simulink library "rewardLibrary"  (R2022b)
settings: Solver=VariableStepAuto  StartTime=0.0  StopTime=10.0  RelTol=1e-3
values from neighbouring files (symbols this model uses):
  accel_vec = (-4:0.5:4)'    [setUpModel.m]
  Ts = 0.1    [setUpMPC.m]
  TsRL = Ts    [setUpRLEnv.m]
  vel_vec = 0:2:20    [setUpModel.m]
undefined symbols (not defined in the file or in its folder): A, B, C, curvature1, D, D_default, DiscIntNeverNeededParam, E, F, gradbp1, k_sigmoid, steer_lim, t_gap, v_set, x_colpen, y_colpen, Z_colpen
libraries: simulink x379, $bdroot x2, mpcadaslib x1
(part 1 of 9)
settings Model: Creator=16koc1  LastModifiedBy=16koc1

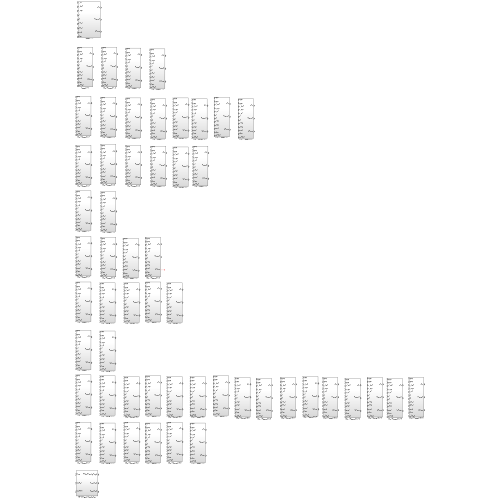
[thumbnail: Simulink's stored preview of the top-level diagram]
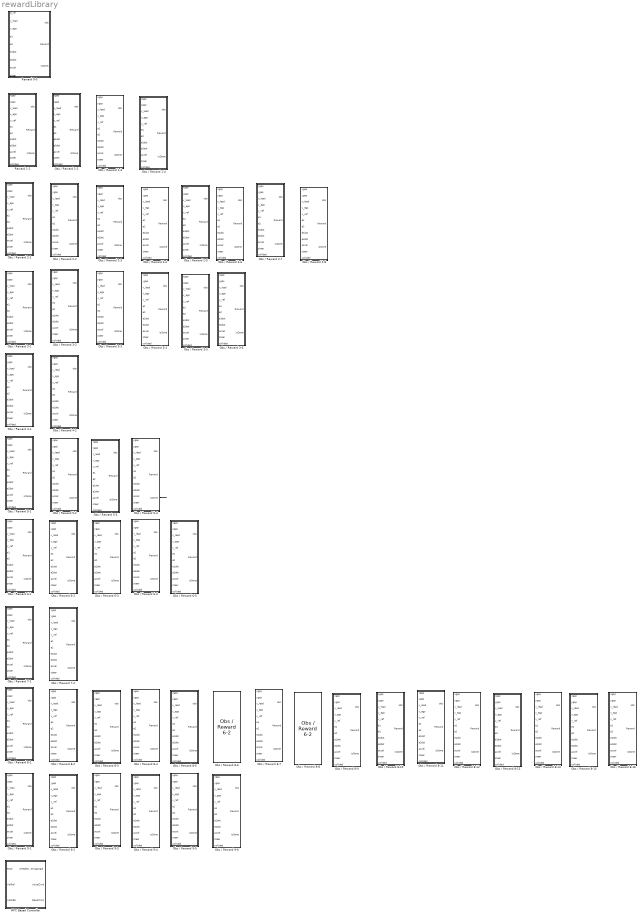
== system rewardLibrary ==
  MPC Based Controller : Subsystem  VariantControl=Stanley
  Obs / Reward 1-2 : Subsystem
  Obs / Reward 1-3 : Subsystem
  Obs / Reward 1-4 : Subsystem
  Obs / Reward 2-1 : Subsystem
  Obs / Reward 2-2 : Subsystem
  Obs / Reward 2-3 : Subsystem
  Obs / Reward 2-4 : Subsystem
  Obs / Reward 2-5 : Subsystem
  Obs / Reward 2-6 : Subsystem
  Obs / Reward 2-7 : Subsystem
  Obs / Reward 2-8 : Subsystem
  Obs / Reward 3-1 : Subsystem
  Obs / Reward 3-2 : Subsystem
  Obs / Reward 3-3 : Subsystem
  Obs / Reward 3-4 : Subsystem
  Obs / Reward 3-5 : Subsystem
  Obs / Reward 3-6 : Subsystem
  Obs / Reward 4-1 : Subsystem
  Obs / Reward 4-2 : Subsystem
  Obs / Reward 5-1 : Subsystem
  Obs / Reward 5-2 : Subsystem
  Obs / Reward 5-3 : Subsystem
  Obs / Reward 5-4 : Subsystem
  Obs / Reward 6-1 : Subsystem  AncestorBlock=rewardLibrary/Obs // Reward 5-3
      settings: LibrarySourceBlock=rewardLibrary/Obs // Reward 5-3
  Obs / Reward 6-2 : Subsystem  AncestorBlock=rewardLibrary/Obs // Reward 5-3
      settings: LibrarySourceBlock=rewardLibrary/Obs // Reward 6-2
  Obs / Reward 6-3 : Subsystem  AncestorBlock=rewardLibrary/Obs // Reward 5-3
      settings: LibrarySourceBlock=rewardLibrary/Obs // Reward 5-3
  Obs / Reward 6-4 : Subsystem  AncestorBlock=rewardLibrary/Obs // Reward 6-2
      settings: LibrarySourceBlock=rewardLibrary/Obs // Reward 6-2
  Obs / Reward 6-5 : Subsystem  AncestorBlock=rewardLibrary/Obs // Reward 6-2
      settings: LibrarySourceBlock=rewardLibrary/Obs // Reward 6-2
  Obs / Reward 7-1 : Subsystem  AncestorBlock=rewardLibrary/Obs // Reward 6-2
      settings: LibrarySourceBlock=rewardLibrary/Obs // Reward 6-2
  Obs / Reward 7-2 : Subsystem  AncestorBlock=rewardLibrary/Obs // Reward 6-2
      settings: LibrarySourceBlock=rewardLibrary/Obs // Reward 6-2
  Obs / Reward 8-1 : Subsystem  AncestorBlock=rewardLibrary/Obs // Reward 6-2
      settings: LibrarySourceBlock=rewardLibrary/Obs // Reward 6-2
  Obs / Reward 8-10 : Subsystem  AncestorBlock=rewardLibrary/Obs // Reward 6-2
      settings: LibrarySourceBlock=rewardLibrary/Obs // Reward 6-2
  Obs / Reward 8-11 : Subsystem  AncestorBlock=rewardLibrary/Obs // Reward 6-2
      settings: LibrarySourceBlock=rewardLibrary/Obs // Reward 6-2
  Obs / Reward 8-12 : Subsystem  AncestorBlock=rewardLibrary/Obs // Reward 6-2
      settings: LibrarySourceBlock=rewardLibrary/Obs // Reward 6-2
  Obs / Reward 8-13 : Subsystem  AncestorBlock=rewardLibrary/Obs // Reward 6-2
      settings: LibrarySourceBlock=rewardLibrary/Obs // Reward 6-2
  Obs / Reward 8-14 : Subsystem  AncestorBlock=rewardLibrary/Obs // Reward 6-2
      settings: LibrarySourceBlock=rewardLibrary/Obs // Reward 6-2
  Obs / Reward 8-15 : Subsystem  AncestorBlock=rewardLibrary/Obs // Reward 6-2
      settings: LibrarySourceBlock=rewardLibrary/Obs // Reward 6-2
  Obs / Reward 8-16 : Subsystem  AncestorBlock=rewardLibrary/Obs // Reward 6-2
      settings: LibrarySourceBlock=rewardLibrary/Obs // Reward 6-2
  Obs / Reward 8-2 : Subsystem  AncestorBlock=rewardLibrary/Obs // Reward 6-2
      settings: LibrarySourceBlock=rewardLibrary/Obs // Reward 6-2
  Obs / Reward 8-3 : Subsystem  AncestorBlock=rewardLibrary/Obs // Reward 6-2
      settings: LibrarySourceBlock=rewardLibrary/Obs // Reward 6-2
  Obs / Reward 8-4 : Subsystem  AncestorBlock=rewardLibrary/Obs // Reward 6-2
      settings: LibrarySourceBlock=rewardLibrary/Obs // Reward 6-2
  Obs / Reward 8-5 : Subsystem  AncestorBlock=rewardLibrary/Obs // Reward 6-2
      settings: LibrarySourceBlock=rewardLibrary/Obs // Reward 6-2
  Obs / Reward 8-6 : $bdroot/Obs // Reward 6-2  SystemSampleTime=-1  VariantActivationTime=update diagram  Latency=0  AutoFrameSizeCalculation=off
  Obs / Reward 8-7 : Subsystem  AncestorBlock=rewardLibrary/Obs // Reward 6-2
      settings: LibrarySourceBlock=rewardLibrary/Obs // Reward 6-2
  Obs / Reward 8-8 : $bdroot/Obs // Reward 6-2  SystemSampleTime=-1  VariantActivationTime=update diagram  Latency=0  AutoFrameSizeCalculation=off
      link override A: Gain=0
      link override Path following/Gain11: Gain=-0.006
      link override Path following/Gain4: Gain=-0.9
  Obs / Reward 8-9 : Subsystem  AncestorBlock=rewardLibrary/Obs // Reward 6-2
      settings: LibrarySourceBlock=rewardLibrary/Obs // Reward 6-2
  Obs / Reward 9-1 : Subsystem  AncestorBlock=rewardLibrary/Obs // Reward 6-2
      settings: LibrarySourceBlock=rewardLibrary/Obs // Reward 6-2
  Obs / Reward 9-2 : Subsystem  AncestorBlock=rewardLibrary/Obs // Reward 6-2
      settings: LibrarySourceBlock=rewardLibrary/Obs // Reward 6-2
  Obs / Reward 9-3 : Subsystem  AncestorBlock=rewardLibrary/Obs // Reward 6-2
      settings: LibrarySourceBlock=rewardLibrary/Obs // Reward 6-2
  Obs / Reward 9-4 : Subsystem  AncestorBlock=rewardLibrary/Obs // Reward 6-2
      settings: LibrarySourceBlock=rewardLibrary/Obs // Reward 6-2
  Obs / Reward 9-5 : Subsystem  AncestorBlock=rewardLibrary/Obs // Reward 6-2
      settings: LibrarySourceBlock=rewardLibrary/Obs // Reward 6-2
  Obs / Reward 9-6 : Subsystem  AncestorBlock=rewardLibrary/Obs // Reward 6-2
      settings: LibrarySourceBlock=rewardLibrary/Obs // Reward 6-2
  Reward 0-0 : Subsystem
  Reward 1-1 : Subsystem
  wires:
  Obs / Reward 5-4/3(isDone) -> ?

== system rewardLibrary/MPC Based Controller ==
  note: This 2-D Lookup Table was created using a for-loop and then normalizing. This is required because the output of the MPC controller is acceleration (m/s^2), but the powertrain model uses pedal commands from 0-1.
      |
      | Here are the steps in the script to create the table:
      |
      | 1.) The for-loop is used to calculate the required torque (Nm) from the powertrain.
      |
      | 2.) The positive torque values are normalized based on peak positive motor torque, and the negative torques are normalized based on the peak brake pressure. This results in a pedal map with values of -1 to 1.
      |
      | This map required two values to be calibrated.
      |
      | This is a simple linearized map, but this can be altered for better drivability.
  note: The 'Dead Zone' blocks is used to ensure that the pedal command is zero.
  note: This block comes from the "Lane Keeping Assist System Using Model Predictive Control" example.
  Pose : Inport
  VelRef : Inport  Port=2
  VelFdbk : Inport  Port=3
  1-D Lookup Table1 : Lookup_n-D  NumberOfTableDimensions=1  BreakpointsForDimension1=gradbp1  Table=curvature1  InterpMethod=Cubic spline  ExtrapMethod=Clip  InternalRulePriority=Speed  RndMeth=Simplest
  Integrator : Integrator
  Path Following Control System MPC : mpcadaslib/Path Following Control System  VariantControl=Variant2  ModelType=Use vehicle parameters  VehicleMass=2000  VehicleYawInertia=4000  LengthToFront=1.4  LengthToRear=1.6  FrontTireStiffness=12e3  RearTireStiffness=11e3  AccelTimeConstant=0.5  EgoModelMatrixA=[-2,zeros(1,3);1,zeros(1,3);zeros(1,2),-4.4021,-12.4603;zeros(1,2),1.3913,-5.1868]  EgoModelMatrixB=[2,zeros(1,3);zeros(1,2),24.1270,15.8609]'  EgoModelMatrixC=[zeros(3,1),eye(3)]  InitialLongVel=v_o1  TransportLag=0  spaceCtrl=off  DefaultSpacing=10  MinSteering=umin  umin_ext=off  MaxSteering=umax  umax_ext=off  MinAcceleration=amin  amin_ext=off  MaxAcceleration=amax  amax_ext=off  Ts=Ts  PredictionHorizon=pred_horizon  ControlHorizon=cont_horizon  LongWeight=w_veltrack  LateralWeight=w_laterror  AccelRateWeight=w_dax  SteerRateWeight=w_dphi  suboptimal=off  maxiter=10  datatypeopt=double  optmode=off  trackmode=off
      link override Longitudinal velocity must be positive: enabled=on
  Pedal map : Subsystem
  Sensor Dynamics : Subsystem
  Terminator : Terminator
  WheelSteeringAngle : Outport
  AccelCmd : Outport  Port=2
  DecelCmd : Outport  Port=3
  wires:
  Integrator/1 -> 1-D Lookup Table1/1
  [ydot1] -> Sensor Dynamics/3(Lateral velocity)
  [yawrate1] -> Sensor Dynamics/4(Yaw rate)
  VelFdbk/1 -> Sensor Dynamics/2(Longitudinal velocity), Path Following Control System MPC/2, Pedal map/1(vx), Integrator/1  "vx"
  VelRef/1 -> Path Following Control System MPC/1
  Pose/1 -> Terminator/1
  Path Following Control System MPC/2 -> WheelSteeringAngle/1
  Path Following Control System MPC/1 -> Pedal map/2(a)  "a"
  Pedal map/1(Out1) -> AccelCmd/1
  Pedal map/2(Out2) -> DecelCmd/1
  Sensor Dynamics/2(Relative yaw angle) -> Path Following Control System MPC/5
  Sensor Dynamics/1(Lateral deviation) -> Path Following Control System MPC/4
  1-D Lookup Table1/1 -> Sensor Dynamics/1(Current curvature), Path Following Control System MPC/3

== system rewardLibrary/Obs // Reward 1-2 ==
  xgap : Inport
  ygap : Inport  Port=2
  v_lead : Inport  Port=3
  v_ego : Inport  Port=4
  v_ref : Inport  Port=5
  e1 : Inport  Port=6
  e2 : Inport  Port=7
  e1dot : Inport  Port=8
  e2dot : Inport  Port=9
  accel : Inport  Port=10
  steer : Inport  Port=11
  collided : Inport  Port=12
  Abs : Abs  SaturateOnIntegerOverflow=off
  Compare To Constant : simulink/Logic and Bit Operations/Compare To Constant  relop=<=  const=6  OutDataTypeStr=boolean
  Gain : Gain  Gain=10
  Subsystem : Subsystem
  Subsystem1 : Subsystem
  Subsystem2 : Subsystem
  Sum : Sum  Inputs=-+|
  Terminator{,1..3} (4 alike) : Terminator
  obs : Outport  VectorParamsAs1DForOutWhenUnconnected=off
  Reward : Outport  Port=2  VectorParamsAs1DForOutWhenUnconnected=off
  isDone : Outport  Port=3  VectorParamsAs1DForOutWhenUnconnected=off
  tag scope: onTrack=global
  wires:
  e2dot/1 -> Subsystem/6(e2dot)
  e1/1 -> Abs/1, Subsystem/3(e1), Subsystem2/2(e1), Subsystem1/2(e1)
  e2/1 -> Subsystem2/3(e2), Subsystem/4(e2)
  v_ego/1 -> Subsystem2/1(v_ego), Subsystem/1(v_ego)
  Subsystem2/1(isDone) -> Gain/1, isDone/1
  Subsystem/2(v_err) -> Subsystem1/3(v_err)
  v_lead/1 -> Terminator/1
  xgap/1 -> Terminator1/1
  steer/1 -> Subsystem1/1(steer)
  Subsystem/1(obs) -> obs/1
  e1dot/1 -> Subsystem/5(e1dot)
  Subsystem1/1(reward) -> Sum/2
  Sum/1 -> Reward/1
  Gain/1 -> Sum/1
  Abs/1 -> Compare To Constant/1
  Compare To Constant/1 -> [onTrack]
  collided/1 -> Terminator3/1
  v_ref/1 -> Subsystem/2(v_ref)
  ygap/1 -> Terminator2/1
  accel/1 -> Subsystem1/4(accel)

== system rewardLibrary/Obs // Reward 1-3 ==
  xgap : Inport
  ygap : Inport  Port=2
  v_lead : Inport  Port=3
  v_ego : Inport  Port=4
  v_ref : Inport  Port=5
  e1 : Inport  Port=6
  e2 : Inport  Port=7
  e1dot : Inport  Port=8
  e2dot : Inport  Port=9
  accel : Inport  Port=10
  steer : Inport  Port=11
  collided : Inport  Port=12
  Abs : Abs  SaturateOnIntegerOverflow=off
  Compare To Constant : simulink/Logic and Bit Operations/Compare To Constant  relop=<=  const=6  OutDataTypeStr=boolean
  Gain : Gain  Gain=300
  Subsystem : Subsystem
  Subsystem1 : Subsystem
  Subsystem2 : Subsystem
  Sum : Sum  Inputs=-+|
  Terminator{,1..3} (4 alike) : Terminator
  obs : Outport  VectorParamsAs1DForOutWhenUnconnected=off
  Reward : Outport  Port=2  VectorParamsAs1DForOutWhenUnconnected=off
  isDone : Outport  Port=3  VectorParamsAs1DForOutWhenUnconnected=off
  tag scope: onTrack=global
  wires:
  e2dot/1 -> Subsystem/6(e2dot)
  e1/1 -> Abs/1, Subsystem/3(e1), Subsystem2/2(e1), Subsystem1/2(e1)
  e2/1 -> Subsystem2/3(e2), Subsystem/4(e2)
  v_ego/1 -> Subsystem2/1(v_ego), Subsystem/1(v_ego)
  Subsystem2/1(isDone) -> Gain/1, isDone/1
  Subsystem/2(v_err) -> Subsystem1/3(v_err)
  v_lead/1 -> Terminator/1
  xgap/1 -> Terminator1/1
  steer/1 -> Subsystem1/1(steer)
  Subsystem/1(obs) -> obs/1
  e1dot/1 -> Subsystem/5(e1dot)
  Subsystem1/1(reward) -> Sum/2
  Sum/1 -> Reward/1
  Gain/1 -> Sum/1
  Abs/1 -> Compare To Constant/1
  Compare To Constant/1 -> [onTrack]
  collided/1 -> Terminator3/1
  v_ref/1 -> Subsystem/2(v_ref)
  ygap/1 -> Terminator2/1
  accel/1 -> Subsystem1/4(accel)

== system rewardLibrary/Obs // Reward 1-4 ==
  xgap : Inport
  ygap : Inport  Port=2
  v_lead : Inport  Port=3
  v_ego : Inport  Port=4
  v_ref : Inport  Port=5
  e1 : Inport  Port=6
  e2 : Inport  Port=7
  e1dot : Inport  Port=8
  e2dot : Inport  Port=9
  accel : Inport  Port=10
  steer : Inport  Port=11
  collided : Inport  Port=12
  Abs : Abs  SaturateOnIntegerOverflow=off
  Compare To Constant : simulink/Logic and Bit Operations/Compare To Constant  relop=<=  const=6  OutDataTypeStr=boolean
  Gain : Gain  Gain=100
  Subsystem : Subsystem
  Subsystem1 : Subsystem
  Subsystem2 : Subsystem
  Sum : Sum  Inputs=-+|
  Terminator{,1..3} (4 alike) : Terminator
  obs : Outport  VectorParamsAs1DForOutWhenUnconnected=off
  Reward : Outport  Port=2  VectorParamsAs1DForOutWhenUnconnected=off
  isDone : Outport  Port=3  VectorParamsAs1DForOutWhenUnconnected=off
  tag scope: onTrack=global
  wires:
  e2dot/1 -> Subsystem/6(e2dot)
  e1/1 -> Abs/1, Subsystem/3(e1), Subsystem2/2(e1), Subsystem1/2(e1)
  e2/1 -> Subsystem2/3(e2), Subsystem/4(e2)
  v_ego/1 -> Subsystem2/1(v_ego), Subsystem/1(v_ego)
  Subsystem2/1(isDone) -> Gain/1, isDone/1
  Subsystem/2(v_err) -> Subsystem1/3(v_err)
  v_lead/1 -> Terminator/1
  xgap/1 -> Terminator1/1
  steer/1 -> Subsystem1/1(steer)
  Subsystem/1(obs) -> obs/1
  e1dot/1 -> Subsystem/5(e1dot)
  Subsystem1/1(reward) -> Sum/2
  Sum/1 -> Reward/1
  Gain/1 -> Sum/1
  Abs/1 -> Compare To Constant/1
  Compare To Constant/1 -> [onTrack]
  collided/1 -> Terminator3/1
  v_ref/1 -> Subsystem/2(v_ref)
  ygap/1 -> Terminator2/1
  accel/1 -> Subsystem1/4(accel)

== system rewardLibrary/Obs // Reward 2-1 ==
  xgap : Inport
  ygap : Inport  Port=2
  v_lead : Inport  Port=3
  v_ego : Inport  Port=4
  v_ref : Inport  Port=5
  e1 : Inport  Port=6
  e2 : Inport  Port=7
  e1dot : Inport  Port=8
  e2dot : Inport  Port=9
  accel : Inport  Port=10
  steer : Inport  Port=11
  collided : Inport  Port=12
  Abs : Abs  SaturateOnIntegerOverflow=off
  Compare To Constant : simulink/Logic and Bit Operations/Compare To Constant  relop=<=  const=6  OutDataTypeStr=boolean
  Gain : Gain  Gain=10
  Subsystem : Subsystem
  Subsystem1 : Subsystem
  Subsystem2 : Subsystem
  Sum : Sum  Inputs=-+|
  Terminator{,1..3} (4 alike) : Terminator
  obs : Outport  VectorParamsAs1DForOutWhenUnconnected=off
  Reward : Outport  Port=2  VectorParamsAs1DForOutWhenUnconnected=off
  isDone : Outport  Port=3  VectorParamsAs1DForOutWhenUnconnected=off
  tag scope: onTrack=global
  wires:
  e2dot/1 -> Subsystem/6(e2dot)
  e1/1 -> Abs/1, Subsystem1/2(e1), Subsystem/3(e1), Subsystem2/2(e1)
  e2/1 -> Subsystem2/3(e2), Subsystem/4(e2)
  v_ego/1 -> Subsystem2/1(v_ego), Subsystem/1(v_ego)
  Subsystem2/1(isDone) -> Gain/1, isDone/1
  v_lead/1 -> Terminator/1
  xgap/1 -> Terminator1/1
  Subsystem/1(obs) -> obs/1
  e1dot/1 -> Subsystem/5(e1dot)
  Sum/1 -> Reward/1
  Gain/1 -> Sum/1
  Abs/1 -> Compare To Constant/1
  Compare To Constant/1 -> [onTrack]
  collided/1 -> Terminator3/1
  v_ref/1 -> Subsystem/2(v_ref)
  ygap/1 -> Terminator2/1
  Subsystem1/1(reward) -> Sum/2
  Subsystem/2(v_err) -> Subsystem1/3(v_err)
  steer/1 -> Subsystem1/1(steer)
  accel/1 -> Subsystem1/4(accel)

== system rewardLibrary/Obs // Reward 2-2 ==
  xgap : Inport
  ygap : Inport  Port=2
  v_lead : Inport  Port=3
  v_ego : Inport  Port=4
  v_ref : Inport  Port=5
  e1 : Inport  Port=6
  e2 : Inport  Port=7
  e1dot : Inport  Port=8
  e2dot : Inport  Port=9
  accel : Inport  Port=10
  steer : Inport  Port=11
  collided : Inport  Port=12
  Abs : Abs  SaturateOnIntegerOverflow=off
  Compare To Constant : simulink/Logic and Bit Operations/Compare To Constant  relop=<=  const=6  OutDataTypeStr=boolean
  Gain : Gain  Gain=10
  Subsystem : Subsystem
  Subsystem1 : Subsystem
  Subsystem2 : Subsystem
  Sum : Sum  Inputs=-+|
  Terminator{,1..3} (4 alike) : Terminator
  obs : Outport  VectorParamsAs1DForOutWhenUnconnected=off
  Reward : Outport  Port=2  VectorParamsAs1DForOutWhenUnconnected=off
  isDone : Outport  Port=3  VectorParamsAs1DForOutWhenUnconnected=off
  tag scope: onTrack=global
  wires:
  e2dot/1 -> Subsystem/6(e2dot)
  e1/1 -> Abs/1, Subsystem1/2(e1), Subsystem/3(e1), Subsystem2/2(e1)
  e2/1 -> Subsystem2/3(e2), Subsystem/4(e2)
  v_ego/1 -> Subsystem2/1(v_ego), Subsystem/1(v_ego)
  Subsystem2/1(isDone) -> Gain/1, isDone/1
  v_lead/1 -> Terminator/1
  xgap/1 -> Terminator1/1
  Subsystem/1(obs) -> obs/1
  e1dot/1 -> Subsystem/5(e1dot)
  Sum/1 -> Reward/1
  Gain/1 -> Sum/1
  Abs/1 -> Compare To Constant/1
  Compare To Constant/1 -> [onTrack]
  collided/1 -> Terminator3/1
  v_ref/1 -> Subsystem/2(v_ref)
  ygap/1 -> Terminator2/1
  Subsystem1/1(reward) -> Sum/2
  Subsystem/2(v_err) -> Subsystem1/3(v_err)
  steer/1 -> Subsystem1/1(steer)
  accel/1 -> Subsystem1/4(accel)

== system rewardLibrary/Obs // Reward 2-3 ==
  xgap : Inport
  ygap : Inport  Port=2
  v_lead : Inport  Port=3
  v_ego : Inport  Port=4
  v_ref : Inport  Port=5
  e1 : Inport  Port=6
  e2 : Inport  Port=7
  e1dot : Inport  Port=8
  e2dot : Inport  Port=9
  accel : Inport  Port=10
  steer : Inport  Port=11
  collided : Inport  Port=12
  Abs : Abs  SaturateOnIntegerOverflow=off
  Compare To Constant : simulink/Logic and Bit Operations/Compare To Constant  relop=<=  const=6  OutDataTypeStr=boolean
  Gain : Gain  Gain=10
  Gain1 : Gain  Gain=100
  OR : Logic  Operator=OR  IconShape=distinctive  AllPortsSameDT=off  OutDataTypeStr=boolean
  Subsystem : Subsystem
  Subsystem1 : Subsystem
  Subsystem2 : Subsystem
  Sum : Sum  Inputs=--+
  Terminator{,1..3} (4 alike) : Terminator
  obs : Outport  VectorParamsAs1DForOutWhenUnconnected=off
  Reward : Outport  Port=2  VectorParamsAs1DForOutWhenUnconnected=off
  isDone : Outport  Port=3  VectorParamsAs1DForOutWhenUnconnected=off
  tag scope: onTrack=global
  wires:
  e2dot/1 -> Subsystem/6(e2dot)
  e1/1 -> Abs/1, Subsystem1/2(e1), Subsystem/3(e1), Subsystem2/2(e1)
  e2/1 -> Subsystem2/3(e2), Subsystem/4(e2)
  v_ego/1 -> Subsystem2/1(v_ego), Subsystem/1(v_ego)
  Subsystem2/1(isDone) -> OR/1, Gain/1
  v_lead/1 -> Terminator/1
  xgap/1 -> Terminator1/1
  Subsystem/1(obs) -> obs/1
  e1dot/1 -> Subsystem/5(e1dot)
  Sum/1 -> Reward/1
  Gain/1 -> Sum/1
  Abs/1 -> Compare To Constant/1
  Compare To Constant/1 -> [onTrack]
  collided/1 -> Terminator3/1
  v_ref/1 -> Subsystem/2(v_ref)
  ygap/1 -> Terminator2/1
  Subsystem1/1(reward) -> Sum/3
  Subsystem/2(v_err) -> Subsystem1/3(v_err)
  steer/1 -> Subsystem1/1(steer)
  accel/1 -> Subsystem1/4(accel)
  OR/1 -> isDone/1
  Subsystem2/2(spinTurn) -> Gain1/1, OR/2
  Gain1/1 -> Sum/2

== system rewardLibrary/Obs // Reward 2-4 ==
  xgap : Inport
  ygap : Inport  Port=2
  v_lead : Inport  Port=3
  v_ego : Inport  Port=4
  v_ref : Inport  Port=5
  e1 : Inport  Port=6
  e2 : Inport  Port=7
  e1dot : Inport  Port=8
  e2dot : Inport  Port=9
  accel : Inport  Port=10
  steer : Inport  Port=11
  collided : Inport  Port=12
  Abs : Abs  SaturateOnIntegerOverflow=off
  Compare To Constant : simulink/Logic and Bit Operations/Compare To Constant  relop=<=  const=6  OutDataTypeStr=boolean
  Gain : Gain  Gain=10
  Gain1 : Gain  Gain=100
  OR : Logic  Operator=OR  IconShape=distinctive  AllPortsSameDT=off  OutDataTypeStr=boolean
  Subsystem : Subsystem
  Subsystem1 : Subsystem
  Subsystem2 : Subsystem
  Sum : Sum  Inputs=--+
  Terminator{,1..3} (4 alike) : Terminator
  obs : Outport  VectorParamsAs1DForOutWhenUnconnected=off
  Reward : Outport  Port=2  VectorParamsAs1DForOutWhenUnconnected=off
  isDone : Outport  Port=3  VectorParamsAs1DForOutWhenUnconnected=off
  tag scope: onTrack=global
  wires:
  e2dot/1 -> Subsystem/6(e2dot)
  e1/1 -> Abs/1, Subsystem1/2(e1), Subsystem/3(e1), Subsystem2/2(e1)
  e2/1 -> Subsystem2/3(e2), Subsystem/4(e2)
  v_ego/1 -> Subsystem2/1(v_ego), Subsystem/1(v_ego)
  Subsystem2/1(isDone) -> OR/1, Gain/1
  v_lead/1 -> Terminator/1
  xgap/1 -> Terminator1/1
  Subsystem/1(obs) -> obs/1
  e1dot/1 -> Subsystem/5(e1dot)
  Sum/1 -> Reward/1
  Gain/1 -> Sum/1
  Abs/1 -> Compare To Constant/1
  Compare To Constant/1 -> [onTrack]
  collided/1 -> Terminator3/1
  v_ref/1 -> Subsystem/2(v_ref)
  ygap/1 -> Terminator2/1
  Subsystem1/1(reward) -> Sum/3
  Subsystem/2(v_err) -> Subsystem1/3(v_err)
  steer/1 -> Subsystem1/1(steer)
  accel/1 -> Subsystem1/4(accel)
  OR/1 -> isDone/1
  Subsystem2/2(spinTurn) -> Gain1/1, OR/2
  Gain1/1 -> Sum/2

== system rewardLibrary/Obs // Reward 2-5 ==
  xgap : Inport
  ygap : Inport  Port=2
  v_lead : Inport  Port=3
  v_ego : Inport  Port=4
  v_ref : Inport  Port=5
  e1 : Inport  Port=6
  e2 : Inport  Port=7
  e1dot : Inport  Port=8
  e2dot : Inport  Port=9
  accel : Inport  Port=10
  steer : Inport  Port=11
  collided : Inport  Port=12
  Abs : Abs  SaturateOnIntegerOverflow=off
  Compare To Constant : simulink/Logic and Bit Operations/Compare To Constant  relop=<=  const=6  OutDataTypeStr=boolean
  Gain : Gain  Gain=10
  Gain1 : Gain  Gain=100
  OR : Logic  Operator=OR  IconShape=distinctive  AllPortsSameDT=off  OutDataTypeStr=boolean
  Subsystem : Subsystem
  Subsystem1 : Subsystem
  Subsystem2 : Subsystem
  Sum : Sum  Inputs=--+
  Terminator{,1..3} (4 alike) : Terminator
  obs : Outport  VectorParamsAs1DForOutWhenUnconnected=off
  Reward : Outport  Port=2  VectorParamsAs1DForOutWhenUnconnected=off
  isDone : Outport  Port=3  VectorParamsAs1DForOutWhenUnconnected=off
  tag scope: onTrack=global
  wires:
  e2dot/1 -> Subsystem/6(e2dot)
  e1/1 -> Abs/1, Subsystem1/2(e1), Subsystem/3(e1), Subsystem2/2(e1)
  e2/1 -> Subsystem2/3(e2), Subsystem/4(e2)
  v_ego/1 -> Subsystem2/1(v_ego), Subsystem/1(v_ego)
  Subsystem2/1(isDone) -> OR/1, Gain/1
  v_lead/1 -> Terminator/1
  xgap/1 -> Terminator1/1
  Subsystem/1(obs) -> obs/1
  e1dot/1 -> Subsystem/5(e1dot)
  Sum/1 -> Reward/1
  Gain/1 -> Sum/1
  Abs/1 -> Compare To Constant/1
  Compare To Constant/1 -> [onTrack]
  collided/1 -> Terminator3/1
  v_ref/1 -> Subsystem/2(v_ref)
  ygap/1 -> Terminator2/1
  Subsystem1/1(reward) -> Sum/3
  Subsystem/2(v_err) -> Subsystem1/3(v_err)
  steer/1 -> Subsystem1/1(steer)
  accel/1 -> Subsystem1/4(accel)
  OR/1 -> isDone/1
  Subsystem2/2(spinTurn) -> Gain1/1, OR/2
  Gain1/1 -> Sum/2

== system rewardLibrary/Obs // Reward 2-6 ==
  xgap : Inport
  ygap : Inport  Port=2
  v_lead : Inport  Port=3
  v_ego : Inport  Port=4
  v_ref : Inport  Port=5
  e1 : Inport  Port=6
  e2 : Inport  Port=7
  e1dot : Inport  Port=8
  e2dot : Inport  Port=9
  accel : Inport  Port=10
  steer : Inport  Port=11
  collided : Inport  Port=12
  Abs : Abs  SaturateOnIntegerOverflow=off
  Compare To Constant : simulink/Logic and Bit Operations/Compare To Constant  relop=<=  const=6  OutDataTypeStr=boolean
  Gain : Gain  Gain=10
  Gain1 : Gain  Gain=100
  OR : Logic  Operator=OR  IconShape=distinctive  AllPortsSameDT=off  OutDataTypeStr=boolean
  Subsystem : Subsystem
  Subsystem1 : Subsystem
  Subsystem2 : Subsystem
  Sum : Sum  Inputs=--+
  Terminator{,1..3} (4 alike) : Terminator
  obs : Outport  VectorParamsAs1DForOutWhenUnconnected=off
  Reward : Outport  Port=2  VectorParamsAs1DForOutWhenUnconnected=off
  isDone : Outport  Port=3  VectorParamsAs1DForOutWhenUnconnected=off
  tag scope: onTrack=global
  wires:
  e2dot/1 -> Subsystem/6(e2dot)
  e1/1 -> Abs/1, Subsystem1/2(e1), Subsystem/3(e1), Subsystem2/2(e1)
  e2/1 -> Subsystem2/3(e2), Subsystem/4(e2)
  v_ego/1 -> Subsystem2/1(v_ego), Subsystem/1(v_ego)
  Subsystem2/1(isDone) -> OR/1, Gain/1
  v_lead/1 -> Terminator/1
  xgap/1 -> Terminator1/1
  Subsystem/1(obs) -> obs/1
  e1dot/1 -> Subsystem/5(e1dot)
  Sum/1 -> Reward/1
  Gain/1 -> Sum/1
  Abs/1 -> Compare To Constant/1
  Compare To Constant/1 -> [onTrack]
  collided/1 -> Terminator3/1
  v_ref/1 -> Subsystem/2(v_ref)
  ygap/1 -> Terminator2/1
  Subsystem1/1(reward) -> Sum/3
  Subsystem/2(v_err) -> Subsystem1/3(v_err)
  steer/1 -> Subsystem1/1(steer)
  accel/1 -> Subsystem1/4(accel)
  OR/1 -> isDone/1
  Subsystem2/2(spinTurn) -> Gain1/1, OR/2
  Gain1/1 -> Sum/2

== system rewardLibrary/Obs // Reward 2-7 ==
  xgap : Inport
  ygap : Inport  Port=2
  v_lead : Inport  Port=3
  v_ego : Inport  Port=4
  v_ref : Inport  Port=5
  e1 : Inport  Port=6
  e2 : Inport  Port=7
  e1dot : Inport  Port=8
  e2dot : Inport  Port=9
  accel : Inport  Port=10
  steer : Inport  Port=11
  collided : Inport  Port=12
  Abs : Abs  SaturateOnIntegerOverflow=off
  Compare To Constant : simulink/Logic and Bit Operations/Compare To Constant  relop=<=  const=6  OutDataTypeStr=boolean
  Gain : Gain  Gain=10
  Gain1 : Gain  Gain=100
  OR : Logic  Operator=OR  IconShape=distinctive  AllPortsSameDT=off  OutDataTypeStr=boolean
  Subsystem : Subsystem
  Subsystem1 : Subsystem
  Subsystem2 : Subsystem
  Sum : Sum  Inputs=--+
  Terminator{,1..3} (4 alike) : Terminator
  obs : Outport  VectorParamsAs1DForOutWhenUnconnected=off
  Reward : Outport  Port=2  VectorParamsAs1DForOutWhenUnconnected=off
  isDone : Outport  Port=3  VectorParamsAs1DForOutWhenUnconnected=off
  tag scope: onTrack=global
  wires:
  e2dot/1 -> Subsystem/6(e2dot)
  e1/1 -> Abs/1, Subsystem1/2(e1), Subsystem/3(e1), Subsystem2/2(e1)
  e2/1 -> Subsystem2/3(e2), Subsystem/4(e2)
  v_ego/1 -> Subsystem2/1(v_ego), Subsystem/1(v_ego)
  Subsystem2/1(isDone) -> OR/1, Gain/1
  v_lead/1 -> Terminator/1
  xgap/1 -> Terminator1/1
  Subsystem/1(obs) -> obs/1
  e1dot/1 -> Subsystem/5(e1dot)
  Sum/1 -> Reward/1
  Gain/1 -> Sum/1
  Abs/1 -> Compare To Constant/1
  Compare To Constant/1 -> [onTrack]
  collided/1 -> Terminator3/1
  v_ref/1 -> Subsystem/2(v_ref)
  ygap/1 -> Terminator2/1
  Subsystem1/1(reward) -> Sum/3
  Subsystem/2(v_err) -> Subsystem1/3(v_err)
  steer/1 -> Subsystem1/1(steer)
  accel/1 -> Subsystem1/4(accel)
  OR/1 -> isDone/1
  Subsystem2/2(spinTurn) -> Gain1/1, OR/2
  Gain1/1 -> Sum/2

== system rewardLibrary/Obs // Reward 2-8 ==
  xgap : Inport
  ygap : Inport  Port=2
  v_lead : Inport  Port=3
  v_ego : Inport  Port=4
  v_ref : Inport  Port=5
  e1 : Inport  Port=6
  e2 : Inport  Port=7
  e1dot : Inport  Port=8
  e2dot : Inport  Port=9
  accel : Inport  Port=10
  steer : Inport  Port=11
  collided : Inport  Port=12
  Abs : Abs  SaturateOnIntegerOverflow=off
  Compare To Constant : simulink/Logic and Bit Operations/Compare To Constant  relop=<=  const=6  OutDataTypeStr=boolean
  Gain : Gain  Gain=10
  Gain1 : Gain  Gain=100
  OR : Logic  Operator=OR  IconShape=distinctive  AllPortsSameDT=off  OutDataTypeStr=boolean
  Subsystem : Subsystem
  Subsystem1 : Subsystem
  Subsystem2 : Subsystem
  Sum : Sum  Inputs=--+
  Terminator{,1..3} (4 alike) : Terminator
  obs : Outport  VectorParamsAs1DForOutWhenUnconnected=off
  Reward : Outport  Port=2  VectorParamsAs1DForOutWhenUnconnected=off
  isDone : Outport  Port=3  VectorParamsAs1DForOutWhenUnconnected=off
  tag scope: onTrack=global
  wires:
  e2dot/1 -> Subsystem/6(e2dot)
  e1/1 -> Abs/1, Subsystem1/2(e1), Subsystem/3(e1), Subsystem2/2(e1)
  e2/1 -> Subsystem2/3(e2), Subsystem/4(e2)
  v_ego/1 -> Subsystem2/1(v_ego), Subsystem/1(v_ego)
  Subsystem2/1(isDone) -> OR/1, Gain/1
  v_lead/1 -> Terminator/1
  xgap/1 -> Terminator1/1
  Subsystem/1(obs) -> obs/1
  e1dot/1 -> Subsystem/5(e1dot)
  Sum/1 -> Reward/1
  Gain/1 -> Sum/1
  Abs/1 -> Compare To Constant/1
  Compare To Constant/1 -> [onTrack]
  collided/1 -> Terminator3/1
  v_ref/1 -> Subsystem/2(v_ref)
  ygap/1 -> Terminator2/1
  Subsystem1/1(reward) -> Sum/3
  Subsystem/2(v_err) -> Subsystem1/3(v_err)
  steer/1 -> Subsystem1/1(steer)
  accel/1 -> Subsystem1/4(accel)
  OR/1 -> isDone/1
  Subsystem2/2(spinTurn) -> Gain1/1, OR/2
  Gain1/1 -> Sum/2

== system rewardLibrary/Obs // Reward 3-1 ==
  xgap : Inport
  ygap : Inport  Port=2
  v_lead : Inport  Port=3
  v_ego : Inport  Port=4
  v_ref : Inport  Port=5
  e1 : Inport  Port=6
  e2 : Inport  Port=7
  e1dot : Inport  Port=8
  e2dot : Inport  Port=9
  accel : Inport  Port=10
  steer : Inport  Port=11
  collided : Inport  Port=12
  Abs : Abs  SaturateOnIntegerOverflow=off
  Compare To Constant : simulink/Logic and Bit Operations/Compare To Constant  relop=<=  const=6  OutDataTypeStr=boolean
  Gain : Gain  Gain=10
  Gain1 : Gain  Gain=100
  OR : Logic  Operator=OR  IconShape=distinctive  AllPortsSameDT=off  OutDataTypeStr=boolean
  Subsystem : Subsystem
  Subsystem1 : Subsystem
  Subsystem2 : Subsystem
  Sum : Sum  Inputs=--+
  Terminator{,1..3} (4 alike) : Terminator
  obs : Outport  VectorParamsAs1DForOutWhenUnconnected=off
  Reward : Outport  Port=2  VectorParamsAs1DForOutWhenUnconnected=off
  isDone : Outport  Port=3  VectorParamsAs1DForOutWhenUnconnected=off
  tag scope: onTrack=global
  wires:
  e2dot/1 -> Subsystem/6(e2dot)
  e1/1 -> Abs/1, Subsystem1/2(e1), Subsystem/3(e1), Subsystem2/2(e1)
  e2/1 -> Subsystem2/3(e2), Subsystem/4(e2)
  v_ego/1 -> Subsystem2/1(v_ego), Subsystem/1(v_ego)
  Subsystem2/1(isDone) -> OR/1, Gain/1
  v_lead/1 -> Terminator/1
  xgap/1 -> Terminator1/1
  Subsystem/1(obs) -> obs/1
  e1dot/1 -> Subsystem/5(e1dot)
  Sum/1 -> Reward/1
  Gain/1 -> Sum/1
  Abs/1 -> Compare To Constant/1
  Compare To Constant/1 -> [onTrack]
  collided/1 -> Terminator3/1
  v_ref/1 -> Subsystem/2(v_ref)
  ygap/1 -> Terminator2/1
  Subsystem1/1(reward) -> Sum/3
  Subsystem/2(v_err) -> Subsystem1/3(v_err)
  steer/1 -> Subsystem1/1(steer)
  accel/1 -> Subsystem1/4(accel)
  OR/1 -> isDone/1
  Subsystem2/2(spinTurn) -> Gain1/1, OR/2
  Gain1/1 -> Sum/2

== system rewardLibrary/Obs // Reward 3-2 ==
  xgap : Inport
  ygap : Inport  Port=2
  v_lead : Inport  Port=3
  v_ego : Inport  Port=4
  v_ref : Inport  Port=5
  e1 : Inport  Port=6
  e2 : Inport  Port=7
  e1dot : Inport  Port=8
  e2dot : Inport  Port=9
  accel : Inport  Port=10
  steer : Inport  Port=11
  collided : Inport  Port=12
  Abs : Abs  SaturateOnIntegerOverflow=off
  Compare To Constant : simulink/Logic and Bit Operations/Compare To Constant  relop=<=  const=6  OutDataTypeStr=boolean
  Gain1 : Gain  Gain=100
  Subsystem : Subsystem
  Subsystem1 : Subsystem
  Subsystem2 : Subsystem
  Sum : Sum  Inputs=-+
  Terminator{,1..3} (4 alike) : Terminator
  obs : Outport  VectorParamsAs1DForOutWhenUnconnected=off
  Reward : Outport  Port=2  VectorParamsAs1DForOutWhenUnconnected=off
  isDone : Outport  Port=3  VectorParamsAs1DForOutWhenUnconnected=off
  tag scope: onTrack=global
  wires:
  e2dot/1 -> Subsystem/6(e2dot)
  e1/1 -> Abs/1, Subsystem1/2(e1), Subsystem/3(e1), Subsystem2/2(e1)
  e2/1 -> Subsystem2/3(e2), Subsystem/4(e2)
  v_ego/1 -> Subsystem2/1(v_ego), Subsystem/1(v_ego)
  v_lead/1 -> Terminator/1
  xgap/1 -> Terminator1/1
  Subsystem/1(obs) -> obs/1
  e1dot/1 -> Subsystem/5(e1dot)
  Sum/1 -> Reward/1
  Gain1/1 -> Sum/1
  Abs/1 -> Compare To Constant/1
  Compare To Constant/1 -> [onTrack]
  collided/1 -> Terminator3/1
  v_ref/1 -> Subsystem/2(v_ref)
  ygap/1 -> Terminator2/1
  Subsystem1/1(reward) -> Sum/2
  Subsystem/2(v_err) -> Subsystem1/3(v_err)
  steer/1 -> Subsystem1/1(steer)
  accel/1 -> Subsystem1/4(accel)
  Subsystem2/1(isDone) -> Gain1/1, isDone/1

== system rewardLibrary/Obs // Reward 3-3 ==
  xgap : Inport
  ygap : Inport  Port=2
  v_lead : Inport  Port=3
  v_ego : Inport  Port=4
  v_ref : Inport  Port=5
  e1 : Inport  Port=6
  e2 : Inport  Port=7
  e1dot : Inport  Port=8
  e2dot : Inport  Port=9
  accel : Inport  Port=10
  steer : Inport  Port=11
  collided : Inport  Port=12
  Abs : Abs  SaturateOnIntegerOverflow=off
  Compare To Constant : simulink/Logic and Bit Operations/Compare To Constant  relop=<=  const=6  OutDataTypeStr=boolean
  Gain1 : Gain  Gain=100
  Subsystem : Subsystem
  Subsystem1 : Subsystem
  Subsystem2 : Subsystem
  Sum : Sum  Inputs=-+
  Terminator{,1..3} (4 alike) : Terminator
  obs : Outport  VectorParamsAs1DForOutWhenUnconnected=off
  Reward : Outport  Port=2  VectorParamsAs1DForOutWhenUnconnected=off
  isDone : Outport  Port=3  VectorParamsAs1DForOutWhenUnconnected=off
  tag scope: onTrack=global
  wires:
  e2dot/1 -> Subsystem/6(e2dot)
  e1/1 -> Abs/1, Subsystem1/2(e1), Subsystem/3(e1), Subsystem2/2(e1)
  e2/1 -> Subsystem2/3(e2), Subsystem/4(e2)
  v_ego/1 -> Subsystem2/1(v_ego), Subsystem/1(v_ego)
  v_lead/1 -> Terminator/1
  xgap/1 -> Terminator1/1
  Subsystem/1(obs) -> obs/1
  e1dot/1 -> Subsystem/5(e1dot)
  Sum/1 -> Reward/1
  Gain1/1 -> Sum/1
  Abs/1 -> Compare To Constant/1
  Compare To Constant/1 -> [onTrack]
  collided/1 -> Terminator3/1
  v_ref/1 -> Subsystem/2(v_ref)
  ygap/1 -> Terminator2/1
  Subsystem1/1(reward) -> Sum/2
  Subsystem/2(v_err) -> Subsystem1/3(v_err)
  steer/1 -> Subsystem1/1(steer)
  accel/1 -> Subsystem1/4(accel)
  Subsystem2/1(isDone) -> Gain1/1, isDone/1

== system rewardLibrary/Obs // Reward 3-4 ==
  xgap : Inport
  ygap : Inport  Port=2
  v_lead : Inport  Port=3
  v_ego : Inport  Port=4
  v_ref : Inport  Port=5
  e1 : Inport  Port=6
  e2 : Inport  Port=7
  e1dot : Inport  Port=8
  e2dot : Inport  Port=9
  accel : Inport  Port=10
  steer : Inport  Port=11
  collided : Inport  Port=12
  Abs : Abs  SaturateOnIntegerOverflow=off
  Compare To Constant : simulink/Logic and Bit Operations/Compare To Constant  relop=<=  const=6  OutDataTypeStr=boolean
  Gain1 : Gain  Gain=100
  Gain2 : Gain  Gain=300
  OR : Logic  Operator=OR  IconShape=distinctive  AllPortsSameDT=off  OutDataTypeStr=boolean
  Subsystem : Subsystem
  Subsystem1 : Subsystem
  Subsystem2 : Subsystem
  Sum : Sum  Inputs=--+
  Terminator{,1..3} (4 alike) : Terminator
  obs : Outport  VectorParamsAs1DForOutWhenUnconnected=off
  Reward : Outport  Port=2  VectorParamsAs1DForOutWhenUnconnected=off
  isDone : Outport  Port=3  VectorParamsAs1DForOutWhenUnconnected=off
  tag scope: onTrack=global
  wires:
  e2dot/1 -> Subsystem/6(e2dot)
  e1/1 -> Abs/1, Subsystem1/2(e1), Subsystem/3(e1), Subsystem2/2(e1)
  e2/1 -> Subsystem2/3(e2), Subsystem/4(e2)
  v_ego/1 -> Subsystem2/1(v_ego), Subsystem/1(v_ego)
  v_lead/1 -> Terminator/1
  xgap/1 -> Terminator1/1
  Subsystem/1(obs) -> obs/1
  e1dot/1 -> Subsystem/5(e1dot)
  Sum/1 -> Reward/1
  Gain1/1 -> Sum/1
  Abs/1 -> Compare To Constant/1
  Compare To Constant/1 -> [onTrack]
  collided/1 -> Terminator3/1
  v_ref/1 -> Subsystem/2(v_ref)
  ygap/1 -> Terminator2/1
  Subsystem1/1(reward) -> Sum/3
  Subsystem/2(v_err) -> Subsystem1/3(v_err)
  steer/1 -> Subsystem1/1(steer)
  accel/1 -> Subsystem1/4(accel)
  Subsystem2/1(isDone) -> OR/1, Gain1/1
  Subsystem2/2(spinTurn) -> OR/2, Gain2/1
  Gain2/1 -> Sum/2
  OR/1 -> isDone/1

== system rewardLibrary/Obs // Reward 3-5 ==
  xgap : Inport
  ygap : Inport  Port=2
  v_lead : Inport  Port=3
  v_ego : Inport  Port=4
  v_ref : Inport  Port=5
  e1 : Inport  Port=6
  e2 : Inport  Port=7
  e1dot : Inport  Port=8
  e2dot : Inport  Port=9
  accel : Inport  Port=10
  steer : Inport  Port=11
  collided : Inport  Port=12
  Abs : Abs  SaturateOnIntegerOverflow=off
  Compare To Constant : simulink/Logic and Bit Operations/Compare To Constant  relop=<=  const=6  OutDataTypeStr=boolean
  Gain1 : Gain  Gain=20
  Gain2 : Gain  Gain=60
  OR : Logic  Operator=OR  IconShape=distinctive  AllPortsSameDT=off  OutDataTypeStr=boolean
  Subsystem : Subsystem
  Subsystem1 : Subsystem
  Subsystem2 : Subsystem
  Sum : Sum  Inputs=--+
  Terminator{,1..3} (4 alike) : Terminator
  obs : Outport  VectorParamsAs1DForOutWhenUnconnected=off
  Reward : Outport  Port=2  VectorParamsAs1DForOutWhenUnconnected=off
  isDone : Outport  Port=3  VectorParamsAs1DForOutWhenUnconnected=off
  tag scope: onTrack=global
  wires:
  e2dot/1 -> Subsystem/6(e2dot)
  e1/1 -> Abs/1, Subsystem1/2(e1), Subsystem/3(e1), Subsystem2/2(e1)
  e2/1 -> Subsystem2/3(e2), Subsystem/4(e2)
  v_ego/1 -> Subsystem2/1(v_ego), Subsystem/1(v_ego)
  v_lead/1 -> Terminator/1
  xgap/1 -> Terminator1/1
  Subsystem/1(obs) -> obs/1
  e1dot/1 -> Subsystem/5(e1dot)
  Sum/1 -> Reward/1
  Gain1/1 -> Sum/1
  Abs/1 -> Compare To Constant/1
  Compare To Constant/1 -> [onTrack]
  collided/1 -> Terminator3/1
  v_ref/1 -> Subsystem/2(v_ref)
  ygap/1 -> Terminator2/1
  Subsystem1/1(reward) -> Sum/3
  Subsystem/2(v_err) -> Subsystem1/3(v_err)
  steer/1 -> Subsystem1/1(steer)
  accel/1 -> Subsystem1/4(accel)
  Subsystem2/1(isDone) -> OR/1, Gain1/1
  Subsystem2/2(spinTurn) -> OR/2, Gain2/1
  Gain2/1 -> Sum/2
  OR/1 -> isDone/1

== system rewardLibrary/Obs // Reward 3-6 ==
  xgap : Inport
  ygap : Inport  Port=2
  v_lead : Inport  Port=3
  v_ego : Inport  Port=4
  v_ref : Inport  Port=5
  e1 : Inport  Port=6
  e2 : Inport  Port=7
  e1dot : Inport  Port=8
  e2dot : Inport  Port=9
  accel : Inport  Port=10
  steer : Inport  Port=11
  collided : Inport  Port=12
  Abs : Abs  SaturateOnIntegerOverflow=off
  Compare To Constant : simulink/Logic and Bit Operations/Compare To Constant  relop=<=  const=6  OutDataTypeStr=boolean
  Gain1 : Gain  Gain=40
  Gain2 : Gain  Gain=200
  Logical Operator1 : Logic  Operator=OR  AllPortsSameDT=off  OutDataTypeStr=boolean
  Subsystem : Subsystem
  Subsystem1 : Subsystem
  Subsystem2 : Subsystem
  Sum : Sum  Inputs=--+
  Terminator{,1..3} (4 alike) : Terminator
  obs : Outport  VectorParamsAs1DForOutWhenUnconnected=off
  Reward : Outport  Port=2  VectorParamsAs1DForOutWhenUnconnected=off
  isDone : Outport  Port=3  VectorParamsAs1DForOutWhenUnconnected=off
  tag scope: onTrack=global
  wires:
  e2dot/1 -> Subsystem/6(e2dot)
  e1/1 -> Abs/1, Subsystem1/2(e1), Subsystem/3(e1), Subsystem2/2(e1)
  e2/1 -> Subsystem2/3(e2), Subsystem/4(e2)
  v_ego/1 -> Subsystem2/1(v_ego), Subsystem/1(v_ego)
  v_lead/1 -> Terminator/1
  xgap/1 -> Terminator1/1
  Subsystem/1(obs) -> obs/1
  e1dot/1 -> Subsystem/5(e1dot)
  Sum/1 -> Reward/1
  Gain1/1 -> Sum/1
  Abs/1 -> Compare To Constant/1
  Compare To Constant/1 -> [onTrack]
  collided/1 -> Terminator3/1
  v_ref/1 -> Subsystem/2(v_ref)
  ygap/1 -> Terminator2/1
  Subsystem1/1(reward) -> Sum/3
  Subsystem/2(v_err) -> Subsystem1/3(v_err)
  steer/1 -> Subsystem1/1(steer)
  accel/1 -> Subsystem1/4(accel)
  Subsystem2/1(offTrack) -> Gain1/1, Logical Operator1/1
  Subsystem2/2(tooSlow / spinTurn) -> Logical Operator1/2, Gain2/1
  Gain2/1 -> Sum/2
  Logical Operator1/1 -> isDone/1

== system rewardLibrary/Obs // Reward 4-1 ==
  xgap : Inport
  ygap : Inport  Port=2
  v_lead : Inport  Port=3
  v_ego : Inport  Port=4
  v_ref : Inport  Port=5
  e1 : Inport  Port=6
  e2 : Inport  Port=7
  e1dot : Inport  Port=8
  e2dot : Inport  Port=9
  accel : Inport  Port=10
  steer : Inport  Port=11
  collided : Inport  Port=12
  Abs : Abs  SaturateOnIntegerOverflow=off
  Compare To Constant : simulink/Logic and Bit Operations/Compare To Constant  relop=<=  const=6  OutDataTypeStr=boolean
  Gain1 : Gain  Gain=10
  Gain2 : Gain  Gain=100
  Logical Operator1 : Logic  Operator=OR  AllPortsSameDT=off  OutDataTypeStr=boolean
  Subsystem : Subsystem
  Subsystem1 : Subsystem
  Subsystem2 : Subsystem
  Sum : Sum  Inputs=--+
  Terminator{,1..3} (4 alike) : Terminator
  obs : Outport  VectorParamsAs1DForOutWhenUnconnected=off
  Reward : Outport  Port=2  VectorParamsAs1DForOutWhenUnconnected=off
  isDone : Outport  Port=3  VectorParamsAs1DForOutWhenUnconnected=off
  tag scope: onTrack=global
  wires:
  e2dot/1 -> Subsystem/6(e2dot)
  e1/1 -> Abs/1, Subsystem1/2(e1), Subsystem/3(e1), Subsystem2/2(e1)
  e2/1 -> Subsystem2/3(e2), Subsystem/4(e2)
  v_ego/1 -> Subsystem2/1(v_ego), Subsystem/1(v_ego)
  v_lead/1 -> Terminator/1
  xgap/1 -> Terminator1/1
  Subsystem/1(obs) -> obs/1
  e1dot/1 -> Subsystem/5(e1dot)
  Sum/1 -> Reward/1
  Gain1/1 -> Sum/1
  Abs/1 -> Compare To Constant/1
  Compare To Constant/1 -> [onTrack]
  collided/1 -> Terminator3/1
  v_ref/1 -> Subsystem/2(v_ref)
  ygap/1 -> Terminator2/1
  Subsystem1/1(reward) -> Sum/3
  Subsystem/2(v_err) -> Subsystem1/3(v_err)
  steer/1 -> Subsystem1/1(steer)
  accel/1 -> Subsystem1/4(accel)
  Subsystem2/1(offTrack) -> Gain1/1, Logical Operator1/1
  Subsystem2/2(tooSlow / spinTurn) -> Logical Operator1/2, Gain2/1
  Gain2/1 -> Sum/2
  Logical Operator1/1 -> isDone/1

== system rewardLibrary/Obs // Reward 4-2 ==
  xgap : Inport
  ygap : Inport  Port=2
  v_lead : Inport  Port=3
  v_ego : Inport  Port=4
  v_ref : Inport  Port=5
  e1 : Inport  Port=6
  e2 : Inport  Port=7
  e1dot : Inport  Port=8
  e2dot : Inport  Port=9
  accel : Inport  Port=10
  steer : Inport  Port=11
  collided : Inport  Port=12
  Abs : Abs  SaturateOnIntegerOverflow=off
  Compare To Constant : simulink/Logic and Bit Operations/Compare To Constant  relop=<=  const=6  OutDataTypeStr=boolean
  Gain1 : Gain  Gain=10
  Gain2 : Gain  Gain=200
  Gain3 : Gain  Gain=100
  Logical Operator1 : Logic  Operator=OR  Inputs=3  AllPortsSameDT=off  OutDataTypeStr=boolean
  Subsystem : Subsystem
  Subsystem1 : Subsystem
  Subsystem2 : Subsystem
  Sum : Sum  Inputs=---+
  Terminator{,1..3} (4 alike) : Terminator
  obs : Outport  VectorParamsAs1DForOutWhenUnconnected=off
  Reward : Outport  Port=2  VectorParamsAs1DForOutWhenUnconnected=off
  isDone : Outport  Port=3  VectorParamsAs1DForOutWhenUnconnected=off
  tag scope: onTrack=global
  wires:
  e2dot/1 -> Subsystem/6(e2dot)
  e1/1 -> Abs/1, Subsystem1/2(e1), Subsystem/3(e1), Subsystem2/2(e1)
  e2/1 -> Subsystem2/3(e2), Subsystem/4(e2)
  v_ego/1 -> Subsystem2/1(v_ego), Subsystem/1(v_ego)
  v_lead/1 -> Terminator/1
  xgap/1 -> Terminator1/1
  Subsystem/1(obs) -> obs/1
  e1dot/1 -> Subsystem/5(e1dot)
  Sum/1 -> Reward/1
  Gain1/1 -> Sum/1
  Abs/1 -> Compare To Constant/1
  Compare To Constant/1 -> [onTrack]
  collided/1 -> Terminator3/1
  v_ref/1 -> Subsystem/2(v_ref)
  ygap/1 -> Terminator2/1
  Subsystem1/1(reward) -> Sum/4
  Subsystem/2(v_err) -> Subsystem1/3(v_err)
  steer/1 -> Subsystem1/1(steer)
  accel/1 -> Subsystem1/4(accel)
  Subsystem2/1(offTrack) -> Gain1/1, Logical Operator1/1
  Subsystem2/2(tooSlow) -> Gain2/1, Logical Operator1/2
  Gain2/1 -> Sum/2
  Logical Operator1/1 -> isDone/1
  Subsystem2/3(spinTurn) -> Gain3/1, Logical Operator1/3
  Gain3/1 -> Sum/3

== system rewardLibrary/Obs // Reward 5-1 ==
  xgap : Inport
  ygap : Inport  Port=2
  v_lead : Inport  Port=3
  v_ego : Inport  Port=4
  v_ref : Inport  Port=5
  e1 : Inport  Port=6
  e2 : Inport  Port=7
  e1dot : Inport  Port=8
  e2dot : Inport  Port=9
  accel : Inport  Port=10
  steer : Inport  Port=11
  collided : Inport  Port=12
  Abs : Abs  SaturateOnIntegerOverflow=off
  Compare To Constant : simulink/Logic and Bit Operations/Compare To Constant  relop=<=  const=6  OutDataTypeStr=boolean
  Gain1 : Gain  Gain=1000
  Gain2 : Gain  Gain=500
  Logical Operator1 : Logic  Operator=OR  AllPortsSameDT=off  OutDataTypeStr=boolean
  Subsystem : Subsystem
  Subsystem1 : Subsystem
  Subsystem2 : Subsystem
  Sum : Sum  Inputs=--+
  Terminator{,1..4} (5 alike) : Terminator
  obs : Outport  VectorParamsAs1DForOutWhenUnconnected=off
  Reward : Outport  Port=2  VectorParamsAs1DForOutWhenUnconnected=off
  isDone : Outport  Port=3  VectorParamsAs1DForOutWhenUnconnected=off
  tag scope: onTrack=global
  wires:
  e2dot/1 -> Subsystem/6(e2dot)
  e1/1 -> Abs/1, Subsystem1/2(e1), Subsystem/3(e1), Subsystem2/2(e1)
  e2/1 -> Subsystem1/3(e2), Subsystem2/3(e2), Subsystem/4(e2)
  v_ego/1 -> Subsystem2/1(v_ego), Subsystem/1(v_ego)
  v_lead/1 -> Terminator/1
  xgap/1 -> Terminator1/1
  Subsystem/1(obs) -> obs/1
  e1dot/1 -> Subsystem/5(e1dot)
  Sum/1 -> Reward/1
  Gain1/1 -> Sum/1
  Abs/1 -> Compare To Constant/1
  Compare To Constant/1 -> [onTrack]
  collided/1 -> Terminator3/1
  v_ref/1 -> Subsystem/2(v_ref)
  ygap/1 -> Terminator2/1
  Subsystem1/1(reward) -> Sum/3
  Subsystem/2(v_err) -> Subsystem1/1(v_err)
  steer/1 -> Subsystem1/4(steer)
  accel/1 -> Subsystem1/5(accel)
  Subsystem2/1(offTrack) -> Gain1/1, Logical Operator1/1
  Subsystem2/2(tooSlow) -> Gain2/1, Logical Operator1/2
  Gain2/1 -> Sum/2
  Logical Operator1/1 -> isDone/1
  Subsystem2/3(spinTurn) -> Terminator4/1

== system rewardLibrary/Obs // Reward 5-2 ==
  xgap : Inport
  ygap : Inport  Port=2
  v_lead : Inport  Port=3
  v_ego : Inport  Port=4
  v_ref : Inport  Port=5
  e1 : Inport  Port=6
  e2 : Inport  Port=7
  e1dot : Inport  Port=8
  e2dot : Inport  Port=9
  accel : Inport  Port=10
  steer : Inport  Port=11
  collided : Inport  Port=12
  Abs : Abs  SaturateOnIntegerOverflow=off
  Compare To Constant : simulink/Logic and Bit Operations/Compare To Constant  relop=<=  const=6  OutDataTypeStr=boolean
  Gain1 : Gain  Gain=20
  Gain2 : Gain  Gain=20
  Gain3 : Gain  Gain=20
  Logical Operator1 : Logic  Operator=OR  Inputs=3  AllPortsSameDT=off  OutDataTypeStr=boolean
  Subsystem : Subsystem
  Subsystem1 : Subsystem
  Subsystem2 : Subsystem
  Sum : Sum  Inputs=---+
  Terminator{,1..3} (4 alike) : Terminator
  obs : Outport  VectorParamsAs1DForOutWhenUnconnected=off
  Reward : Outport  Port=2  VectorParamsAs1DForOutWhenUnconnected=off
  isDone : Outport  Port=3  VectorParamsAs1DForOutWhenUnconnected=off
  tag scope: onTrack=global
  wires:
  e2dot/1 -> Subsystem/6(e2dot)
  e1/1 -> Abs/1, Subsystem1/2(e1), Subsystem/3(e1), Subsystem2/2(e1)
  e2/1 -> Subsystem1/3(e2), Subsystem2/3(e2), Subsystem/4(e2)
  v_ego/1 -> Subsystem2/1(v_ego), Subsystem/1(v_ego)
  v_lead/1 -> Terminator/1
  xgap/1 -> Terminator1/1
  Subsystem/1(obs) -> obs/1
  e1dot/1 -> Subsystem/5(e1dot)
  Sum/1 -> Reward/1
  Gain1/1 -> Sum/1
  Abs/1 -> Compare To Constant/1
  Compare To Constant/1 -> [onTrack]
  collided/1 -> Terminator3/1
  v_ref/1 -> Subsystem/2(v_ref)
  ygap/1 -> Terminator2/1
  Subsystem1/1(reward) -> Sum/4
  Subsystem/2(v_err) -> Subsystem1/1(v_err)
  steer/1 -> Subsystem1/4(steer)
  accel/1 -> Subsystem1/5(accel)
  Subsystem2/1(offTrack) -> Gain1/1, Logical Operator1/1
  Subsystem2/2(tooSlow) -> Gain2/1, Logical Operator1/2
  Gain2/1 -> Sum/2
  Logical Operator1/1 -> isDone/1
  Subsystem2/3(spinTurn) -> Gain3/1, Logical Operator1/3
  Gain3/1 -> Sum/3

== system rewardLibrary/Obs // Reward 5-3 ==
  xgap : Inport
  ygap : Inport  Port=2
  v_lead : Inport  Port=3
  v_ego : Inport  Port=4
  v_ref : Inport  Port=5
  e1 : Inport  Port=6
  e2 : Inport  Port=7
  e1dot : Inport  Port=8
  e2dot : Inport  Port=9
  accel : Inport  Port=10
  steer : Inport  Port=11
  collided : Inport  Port=12
  Abs : Abs  SaturateOnIntegerOverflow=off
  Compare To Constant : simulink/Logic and Bit Operations/Compare To Constant  relop=<=  const=6  OutDataTypeStr=boolean
  Gain1 : Gain  Gain=20
  Gain2 : Gain  Gain=1500
  Logical Operator1 : Logic  Operator=OR  AllPortsSameDT=off  OutDataTypeStr=boolean
  Subsystem : Subsystem
  Subsystem1 : Subsystem
  Subsystem2 : Subsystem
  Sum : Sum  Inputs=-++
  Terminator{,1..3} (4 alike) : Terminator
  obs : Outport  VectorParamsAs1DForOutWhenUnconnected=off
  Reward : Outport  Port=2  VectorParamsAs1DForOutWhenUnconnected=off
  isDone : Outport  Port=3  VectorParamsAs1DForOutWhenUnconnected=off
  tag scope: onTrack=global
  wires:
  e2dot/1 -> Subsystem/6(e2dot)
  e1/1 -> Abs/1, Subsystem1/2(e1), Subsystem/3(e1), Subsystem2/2(e1)
  e2/1 -> Subsystem1/3(e2), Subsystem2/3(e2), Subsystem/4(e2)
  v_lead/1 -> Terminator/1
  xgap/1 -> Terminator1/1
  Subsystem/1(obs) -> obs/1
  e1dot/1 -> Subsystem/5(e1dot)
  Sum/1 -> Reward/1
  Gain1/1 -> Sum/1
  Abs/1 -> Compare To Constant/1
  Compare To Constant/1 -> [onTrack]
  collided/1 -> Terminator3/1
  v_ref/1 -> Subsystem/2(v_ref)
  ygap/1 -> Terminator2/1
  Subsystem1/1(reward) -> Sum/3
  Subsystem/2(v_err) -> Subsystem1/1(v_err)
  steer/1 -> Subsystem1/4(steer)
  accel/1 -> Subsystem1/5(accel)
  Logical Operator1/1 -> isDone/1
  v_ego/1 -> Subsystem2/1(v_ego), Subsystem/1(v_ego)
  Subsystem2/1(fail) -> Gain1/1, Logical Operator1/1
  Subsystem2/2(success) -> Logical Operator1/2, Gain2/1
  Gain2/1 -> Sum/2

== system rewardLibrary/Obs // Reward 5-4 ==
  xgap : Inport
  ygap : Inport  Port=2
  v_lead : Inport  Port=3
  v_ego : Inport  Port=4
  v_ref : Inport  Port=5
  e1 : Inport  Port=6
  e2 : Inport  Port=7
  e1dot : Inport  Port=8
  e2dot : Inport  Port=9
  accel : Inport  Port=10
  steer : Inport  Port=11
  collided : Inport  Port=12
  Abs : Abs  SaturateOnIntegerOverflow=off
  Compare To Constant : simulink/Logic and Bit Operations/Compare To Constant  relop=<=  const=6  OutDataTypeStr=boolean
  Gain1 : Gain  Gain=20
  Gain2 : Gain  Gain=1500
  Logical Operator1 : Logic  Operator=OR  AllPortsSameDT=off  OutDataTypeStr=boolean
  Subsystem : Subsystem
  Subsystem1 : Subsystem
  Subsystem2 : Subsystem
  Sum : Sum  Inputs=-++
  Terminator{,1..3} (4 alike) : Terminator
  obs : Outport  VectorParamsAs1DForOutWhenUnconnected=off
  Reward : Outport  Port=2  VectorParamsAs1DForOutWhenUnconnected=off
  isDone : Outport  Port=3  VectorParamsAs1DForOutWhenUnconnected=off
  tag scope: onTrack=global
  wires:
  e2dot/1 -> Subsystem/6(e2dot)
  e1/1 -> Abs/1, Subsystem1/2(e1), Subsystem/3(e1), Subsystem2/2(e1)
  e2/1 -> Subsystem1/3(e2), Subsystem2/3(e2), Subsystem/4(e2)
  v_lead/1 -> Terminator/1
  xgap/1 -> Terminator1/1
  Subsystem/1(obs) -> obs/1
  e1dot/1 -> Subsystem/5(e1dot)
  Sum/1 -> Reward/1
  Gain1/1 -> Sum/1
  Abs/1 -> Compare To Constant/1
  Compare To Constant/1 -> [onTrack]
  collided/1 -> Terminator3/1
  v_ref/1 -> Subsystem/2(v_ref)
  ygap/1 -> Terminator2/1
  Subsystem1/1(reward) -> Sum/3
  Subsystem/2(v_err) -> Subsystem1/1(v_err)
  steer/1 -> Subsystem1/4(steer)
  accel/1 -> Subsystem1/5(accel)
  Logical Operator1/1 -> isDone/1
  v_ego/1 -> Subsystem2/1(v_ego), Subsystem/1(v_ego)
  Subsystem2/1(fail) -> Gain1/1, Logical Operator1/1
  Subsystem2/2(success) -> Logical Operator1/2, Gain2/1
  Gain2/1 -> Sum/2
